simulink model "Nonlinear_Inverted_Pendulum_Digital"  (R2012b)
settings: Solver=ode5  StartTime=0.0  StopTime=STOP  FixedStep=T  RelTol=1e-3
values from neighbouring files (symbols this model uses):
  B = 0.1    [Nonlinear_Inverted_Pendulum_Digital_m.m]
  g = 9.8    [Nonlinear_Inverted_Pendulum_Digital_m.m]
  I = 0.006    [Nonlinear_Inverted_Pendulum_Digital_m.m]
  K = 365    [Nonlinear_Inverted_Pendulum_Digital_m.m]
  L = 0.3    [Nonlinear_Inverted_Pendulum_Digital_m.m]
  m = 0.2    [Nonlinear_Inverted_Pendulum_Digital_m.m]
  M = 0.5    [Nonlinear_Inverted_Pendulum_Digital_m.m]
  thetaInit = 1    [Nonlinear_Inverted_Pendulum_Digital_m.m]
undefined symbols (not defined in the file or in its folder): dDen, dNum
settings Model: Creator=Andrew  LastModifiedBy=Andrew

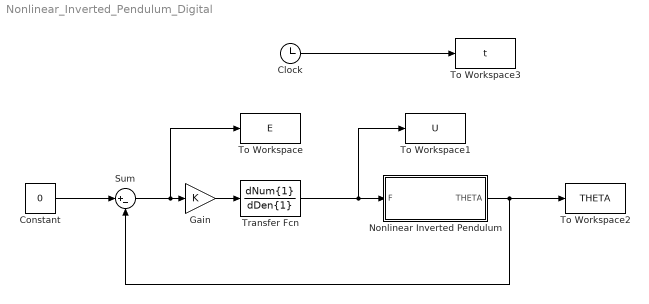
== system Nonlinear_Inverted_Pendulum_Digital ==
  Clock : Clock
  Constant : Constant  Value=0
  Gain : Gain  Gain=K
  Nonlinear Inverted Pendulum : Subsystem
  Sum : Sum  Inputs=|+-
  To Workspace : ToWorkspace  VariableName=E  SampleTime=-1
  To Workspace1 : ToWorkspace  VariableName=U  SampleTime=-1
  To Workspace2 : ToWorkspace  VariableName=THETA  SampleTime=-1
  To Workspace3 : ToWorkspace  VariableName=t  SampleTime=-1
  Transfer Fcn : TransferFcn  Numerator=dNum{1}  Denominator=dDen{1}
  wires:
  Sum/1 -> To Workspace/1, Gain/1
  Nonlinear Inverted Pendulum/1(THETA) -> To Workspace2/1, Sum/2
  Constant/1 -> Sum/1
  Clock/1 -> To Workspace3/1
  Gain/1 -> Transfer Fcn/1
  Transfer Fcn/1 -> Nonlinear Inverted Pendulum/1(F), To Workspace1/1

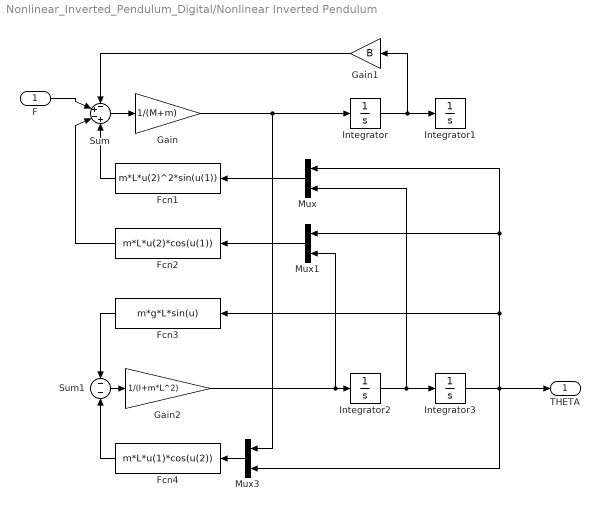
== system Nonlinear_Inverted_Pendulum_Digital/Nonlinear Inverted Pendulum ==
  F : Inport
  Fcn1 : Fcn  Expr=m*L*u(2)^2*sin(u(1))
  Fcn2 : Fcn  Expr=m*L*u(2)*cos(u(1))
  Fcn3 : Fcn  Expr=m*g*L*sin(u)
  Fcn4 : Fcn  Expr=m*L*u(1)*cos(u(2))
  Gain : Gain  Gain=1/(M+m)
  Gain1 : Gain  Gain=B
  Gain2 : Gain  Gain=1/(I+m*L^2)
  Integrator : Integrator
  Integrator1 : Integrator
  Integrator2 : Integrator
  Integrator3 : Integrator  InitialCondition=thetaInit
  Mux : Mux  Inputs=2
  Mux1 : Mux  Inputs=2
  Mux3 : Mux  Inputs=2
  Sum : Sum  Inputs=-+-+
  Sum1 : Sum  Inputs=--
  THETA : Outport
  wires:
  Integrator/1 -> Integrator1/1, Gain1/1
  F/1 -> Sum/2
  Sum/1 -> Gain/1
  Gain/1 -> Mux3/1, Integrator/1
  Gain1/1 -> Sum/1
  Integrator2/1 -> Integrator3/1, Mux/2
  Mux/1 -> Fcn1/1
  Fcn1/1 -> Sum/4
  Mux1/1 -> Fcn2/1
  Fcn2/1 -> Sum/3
  Gain2/1 -> Mux1/2, Integrator2/1
  Sum1/1 -> Gain2/1
  Mux3/1 -> Fcn4/1
  Fcn4/1 -> Sum1/2
  Fcn3/1 -> Sum1/1
  Integrator3/1 -> THETA/1, Mux3/2, Mux1/1, Mux/1, Fcn3/1
